simulink model "SSB_PhaseShiftMethod"  (R2021a)
settings: Solver=VariableStepAuto  StartTime=0.0  StopTime=10.0  RelTol=1e-3
libraries: dspfdesign x1
settings Model: Creator=ZephyrY  LastModifiedBy=ZephyrY

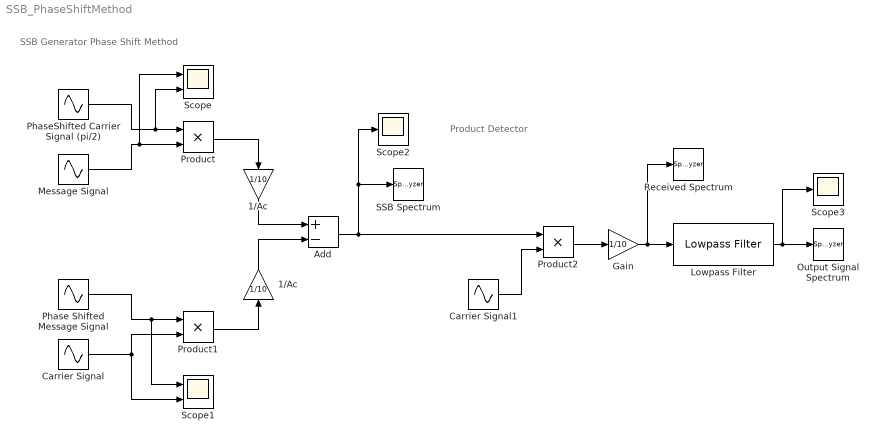
== system SSB_PhaseShiftMethod ==
  note: Product Detector
  note: SSB Generator
      | Phase Shift Method
  1/Ac : Gain  Gain=1/10
  "1/Ac " : Gain  Gain=1/10
  Add : Sum  Inputs=+-
  Carrier Signal : Sin  Amplitude=10  Frequency=2*pi*100  Phase=pi/2  SampleTime=1e-3
  Carrier Signal1 : Sin  Amplitude=10  Frequency=2*pi*100  Phase=pi/2  SampleTime=1e-3
  Gain : Gain  Gain=1/10
  Lowpass Filter : dspfdesign/Lowpass Filter  FilterType=FIR  DesignForMinimumOrder=off  FilterOrder=50  PassbandFrequency=15  StopbandFrequency=12e3  PassbandRipple=0.1  StopbandAttenuation=80  InheritSampleRate=on  SampleRate=44100  SimulateUsing=Interpreted execution  roundingMode=Floor  coeffsDataTypeStr=fixdt(1,16)
  Message Signal : Sin  Amplitude=5  Frequency=2*pi*10  Phase=pi/2  SampleTime=1e-3
  Output Signal Spectrum : SpectrumAnalyzer
  Phase Shifted Message Signal : Sin  Amplitude=5  Frequency=2*pi*10  Phase=pi  SampleTime=1e-3
  PhaseShifted Carrier Signal (pi/2) : Sin  Amplitude=10  Frequency=2*pi*100  Phase=pi  SampleTime=1e-3
  Product : Product
  Product1 : Product
  Product2 : Product
  Received Spectrum : SpectrumAnalyzer
  SSB Spectrum : SpectrumAnalyzer
  Scope : Scope  NumInputPorts=2
  Scope1 : Scope  NumInputPorts=2
  Scope2 : Scope
  Scope3 : Scope
  wires:
  PhaseShifted Carrier Signal (pi/2)/1 -> Scope/2, Product/1
  Message Signal/1 -> Scope/1, Product/2
  Carrier Signal/1 -> Scope1/2, Product1/2
  Product1/1 -> "1/Ac "/1
  Product/1 -> 1/Ac/1
  1/Ac/1 -> Add/1
  "1/Ac "/1 -> Add/2
  Phase Shifted Message Signal/1 -> Scope1/1, Product1/1
  Carrier Signal1/1 -> Product2/2
  Add/1 -> Product2/1, SSB Spectrum/1, Scope2/1
  Product2/1 -> Gain/1
  Gain/1 -> Lowpass Filter/1, Received Spectrum/1
  Lowpass Filter/1 -> Scope3/1, Output Signal Spectrum/1
